simulink library "alphaBeta_ul"  (R2018b)
settings: Solver=VariableStepAuto  StartTime=0.0  StopTime=10.0  RelTol=1e-3
settings Model: Creator=mcobb  LastModifiedBy=asiddiq2

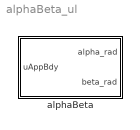
== system alphaBeta_ul ==
  alphaBeta : Subsystem

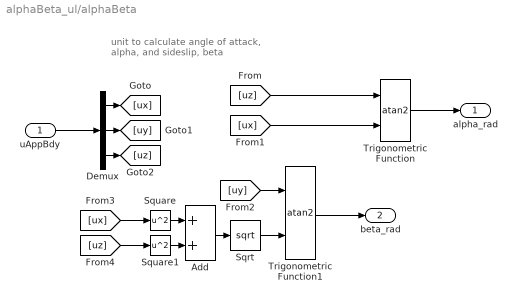
== system alphaBeta_ul/alphaBeta ==
  note: unit to calculate angle of attack,
      | alpha, and sideslip, beta
  uAppBdy : Inport
  Add : Sum
  Demux : Demux  Outputs=3
  Sqrt : Sqrt  SaturateOnIntegerOverflow=on
  Square : Math  Operator=square  SaturateOnIntegerOverflow=on
  Square1 : Math  Operator=square  SaturateOnIntegerOverflow=on
  Trigonometric Function : Trigonometry  Operator=atan2
  Trigonometric Function1 : Trigonometry  Operator=atan2
  alpha_rad : Outport
  beta_rad : Outport  Port=2
  wires:
  uAppBdy/1 -> Demux/1
  Demux/1 -> [ux]
  Demux/2 -> [uy]
  Demux/3 -> [uz]
  [ux] -> Trigonometric Function/2
  Trigonometric Function/1 -> alpha_rad/1
  Trigonometric Function1/1 -> beta_rad/1
  [uy] -> Trigonometric Function1/1
  Square/1 -> Add/1
  Square1/1 -> Add/2
  Add/1 -> Sqrt/1
  [uz] -> Square1/1
  [ux] -> Square/1
  Sqrt/1 -> Trigonometric Function1/2
  [uz] -> Trigonometric Function/1
